simulink model "DCmotor"  (Simulink 8.0)
settings: Solver=ode45  StartTime=0.0  StopTime=50  RelTol=1e-3
settings Model: Creator=dreossi  LastModifiedBy=minopoli
settings DataIOCC: SaveFinalState=on
settings DebuggingCC: SolverPrmCheckMsg=none  InitInArrayFormatMsg=none

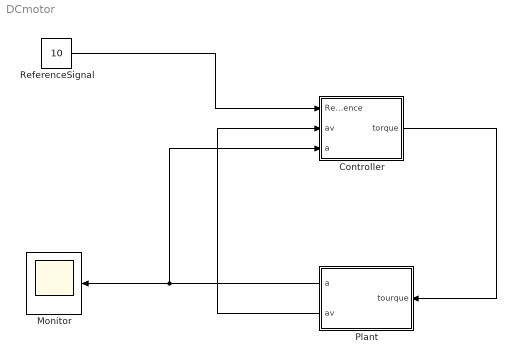
== system DCmotor ==
  Controller : Subsystem
  Monitor : Scope
  Plant : Subsystem
  ReferenceSignal : Constant  Value=10
  wires:
  Controller/1(torque) -> Plant/1(tourque)
  Plant/1(a) -> Monitor/1, Controller/3(a)
  Plant/2(av) -> Controller/2(av)
  ReferenceSignal/1 -> Controller/1(Reference)

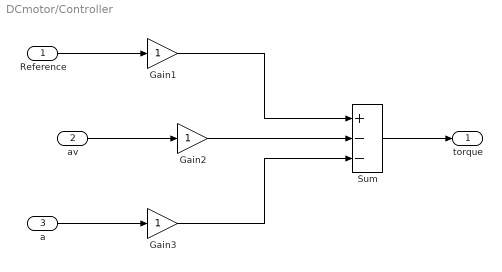
== system DCmotor/Controller ==
  Reference : Inport
  av : Inport  Port=2
  a : Inport  Port=3
  Gain1 : Gain
  Gain2 : Gain
  Gain3 : Gain
  Sum : Sum  Inputs=+--
  torque : Outport
  wires:
  Reference/1 -> Gain1/1
  Sum/1 -> torque/1
  av/1 -> Gain2/1
  a/1 -> Gain3/1
  Gain3/1 -> Sum/3
  Gain1/1 -> Sum/1
  Gain2/1 -> Sum/2

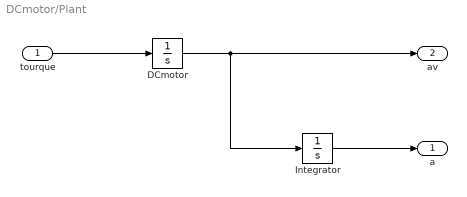
== system DCmotor/Plant ==
  tourque : Inport
  DCmotor : Integrator
  Integrator : Integrator
  a : Outport
  av : Outport  Port=2
  wires:
  tourque/1 -> DCmotor/1
  Integrator/1 -> a/1
  DCmotor/1 -> Integrator/1, av/1
